simulink model "StateflowOnramp"  (R2021a)
settings: Solver=VariableStepAuto  StartTime=0.0  StopTime=10.0  RelTol=1e-3
StartFcn:
  | learning.simulink.modelCallbacks.startFunction(gcs)
StopFcn:
  | learning.simulink.modelCallbacks.stopFunction(gcs)
model workspace (MAT data in the model file):
  courseObject.course = 'stateflow'
  courseObject.chapter = 3
  courseObject.lesson = 2
  courseObject.section = 1
  courseObject.task = 1
libraries: SignalEditorBlockLib x1, signalChecks x1
CloseFcn:
  | learning.simulink.cleanupOnlineTraining
settings Model: Creator=pc  LastModifiedBy=pc
settings DataIOCC: SaveTime=off

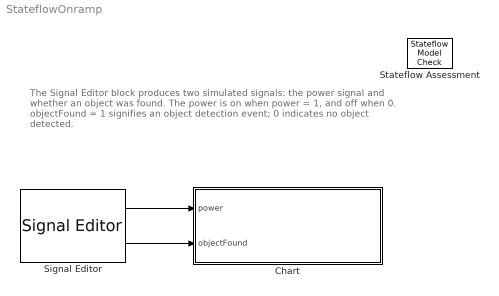
== system StateflowOnramp ==
  note: The Signal Editor block produces two simulated signals: the power signal and whether an object was found.
      | The power is on when power = 1, and off when 0.
      | objectFound = 1 signifies an object detection event; 0 indicates no object detected.
  Chart : Stateflow chart  TreatAsAtomicUnit=on
  Signal Editor : SignalEditorBlockLib/Signal Editor  FileName=objectTrackerTestSignal.mat  ActiveScenario=Scenario  ActiveSignal=Power  IsBus=off  OutputBusObjectStr=Bus: BusObject  SampleTime=0.5  Interpolate=off  ZeroCross=off  OutputAfterFinalValue=Setting to zero  Unit=inherit  PreserveSignalName=on
  Stateflow Assessment : signalChecks/Stateflow Model Check  mlfunc='LearningApplication.gradeStateflowTask'  flags='transitionExOrder'  startInChart=true  lesson=0  task=6  pass=-1
      settings: AttributesFormatString=|
      | No input required
      | for this task
  wires:
  Signal Editor/2 -> Chart/2(objectFound)
  Signal Editor/1 -> Chart/1(power)

== stateflow chart StateflowOnramp/Chart ==
  state Seeking
  state Tracking
  state Off
  (default) -> Off
  Seeking -> Off [order 1] : [power==0]
  Seeking -> Tracking [order 2] : [objectFound==1]
  Off -> Seeking : [power==1]
  Tracking -> Seeking [order 2] : [objectFound==0]
  Tracking -> Off [order 1] : [power==0]
  data: power input; objectFound input
